simulink model "water_tank_model"  (R2024a)
settings: Solver=FixedStepAuto  StartTime=0.0  StopTime=10^7  FixedStep=Ts  RelTol=1e-3
values from neighbouring files (symbols this model uses):
  a1 = 1.31e-4    (= 0.000131)    [init_param.m]    (also in new_algo.m = a1 / scale; plots_thesis.m = a(1))
  a2 = 1.51e-4    (= 0.000151)    [init_param.m]    (also in new_algo.m = a2 / scale; plots_thesis.m = a(2))
  a3 = 9.27e-5    (= 9.27e-05)    [init_param.m]
  a4 = 8.82e-5    (= 8.82e-05)    [init_param.m]
  g = 9.81    [init_param.m]
  ga = 0.30    (= 0.3)    [init_param.m]
  gb = 0.40    (= 0.4)    [init_param.m]
  S = S + x*x.'    [covariance_matrix_calc.m]    (also in init_param.m = 0.06)
settings Model: Creator=phili  LastModifiedBy=phili

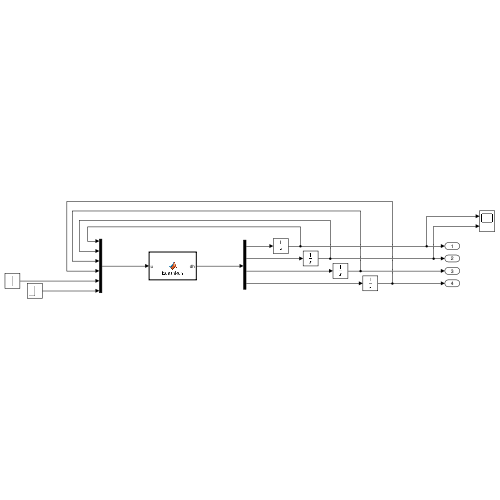
[thumbnail: Simulink's stored preview of the top-level diagram]
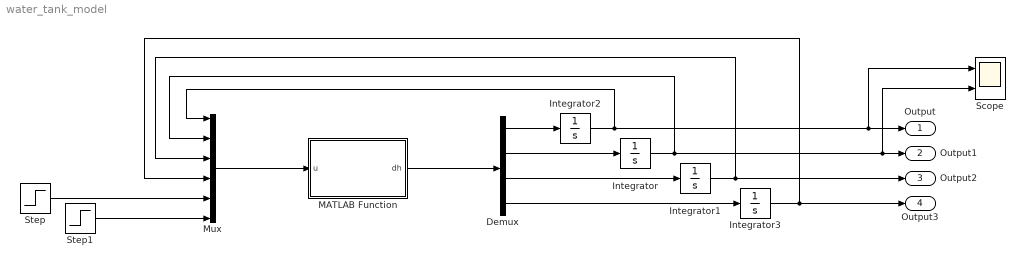
== system water_tank_model ==
  Demux : Demux
  Integrator{,1..3} (4 alike) : Integrator
  MATLAB Function : MATLAB Function  TreatAsAtomicUnit=on
  Mux : Mux  Inputs=6
  Scope : Scope  NumInputPorts=2
  Step : Step  Time=0.0009056  SampleTime=0
  Step1 : Step  Time=0.0011111  SampleTime=0
  Output : Outport
  Output1 : Outport  Port=2
  Output2 : Outport  Port=3
  Output3 : Outport  Port=4
  wires:
  MATLAB Function/1(dh) -> Demux/1
  Mux/1 -> MATLAB Function/1(u)
  Demux/1 -> Integrator2/1
  Demux/2 -> Integrator/1
  Demux/3 -> Integrator1/1
  Demux/4 -> Integrator3/1
  Integrator2/1 -> Scope/1, Output/1, Mux/1
  Integrator/1 -> Scope/2, Output1/1, Mux/2
  Integrator1/1 -> Mux/3, Output2/1
  Integrator3/1 -> Output3/1, Mux/4
  Step/1 -> Mux/5
  Step1/1 -> Mux/6

== matlab function water_tank_model/MATLAB Function ==
  data: u input; dh output; a1 parameter; a2 parameter; a3 parameter; a4 parameter; S parameter; ga parameter; gb parameter; g parameter
function dh = fourtankfun(u, a1, a2, a3, a4, S, ga, gb, g)

h1 = u(1);
h2 = u(2);
h3 = u(3);
h4 = u(4);
qa = u(5);
qb = u(6);

dh1 = (-a1/S)*((2*g*h1)^(1/2)) + (a3/S)*((2*g*h3)^(1/2)) + (ga/S)*qa;
dh2 = (-a2/S)*((2*g*h2)^(1/2)) + (a4/S)*((2*g*h4)^(1/2)) + (gb/S)*qb;
dh3 = (-a3/S)*((2*g*h3)^(1/2)) + ((1-gb)/S)*qb;
dh4 = (-a4/S)*((2*g*h4)^(1/2)) + ((1-ga)/S)*qa;

dh = [dh1; dh2; dh3; dh4];
end
